simulink model "exampleMinRunTime3"  (Simulink 7.6)
settings: Solver=ode45  StartTime=0.0  StopTime=30  RelTol=1e-3
undefined symbols (not defined in the file): minruntime
libraries: simulink x1
settings Model: Creator=drhf  LastModifiedBy=drhf

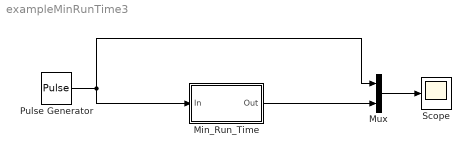
== system exampleMinRunTime3 ==
  Min_Run_Time : Subsystem
  Mux : Mux  Inputs=2
  Pulse Generator : DiscretePulseGenerator  PulseType=Time based  Amplitude=2  Period=10  PulseWidth=5
  Scope : Scope
  wires:
  Pulse Generator/1 -> Mux/1, Min_Run_Time/1(In)
  Mux/1 -> Scope/1
  Min_Run_Time/1(Out) -> Mux/2

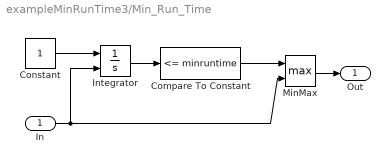
== system exampleMinRunTime3/Min_Run_Time ==
  In : Inport
  Compare To Constant : simulink/Logic and Bit Operations/Compare To Constant  SystemSampleTime=-1  relop=<=  const=minruntime  LogicOutDataTypeMode=uint8
  Constant : Constant
  Integrator : Integrator  ExternalReset=rising
  MinMax : MinMax  Function=max  Inputs=2
  Out : Outport
  wires:
  Constant/1 -> Integrator/1
  Integrator/1 -> Compare To Constant/1
  MinMax/1 -> Out/1
  In/1 -> Integrator/2, MinMax/2
  Compare To Constant/1 -> MinMax/1
